simulink model "model"  (R2016b)
settings: Solver=VariableStepAuto  StartTime=0.0  StopTime=4  RelTol=1e-3
undefined symbols (not defined in the file): k1, k2, k_pd, k_pp, k_rp
settings Model: Creator=Kevin K. Kaldvansvik  LastModifiedBy=Kevin K. Kaldvansvik

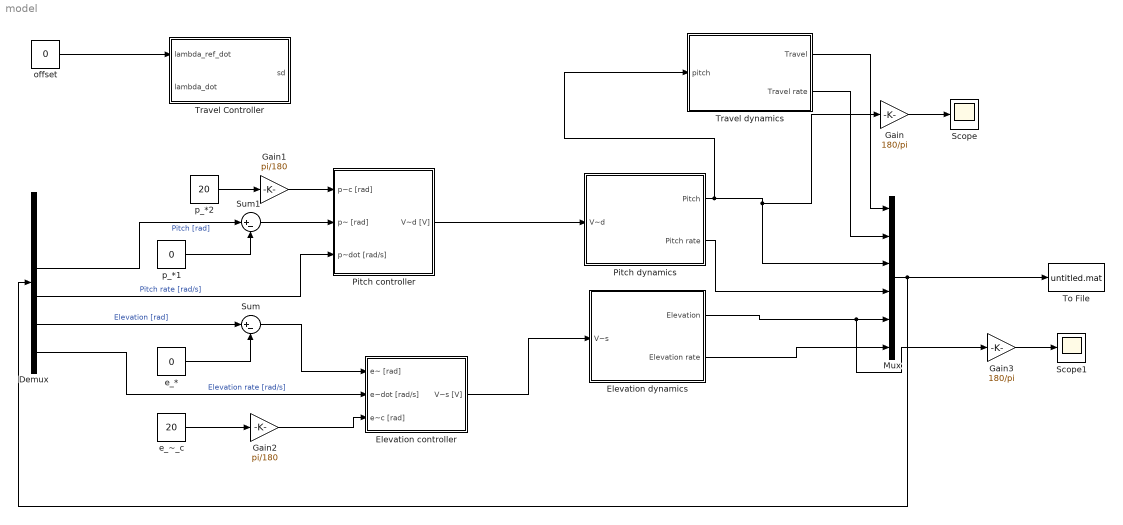
== system model ==
  Demux : Demux  Outputs=6
  Elevation controller : Subsystem
  Elevation dynamics : Subsystem
  Gain : Gain  Gain=180/pi
  Gain1 : Gain  Gain=pi/180
  Gain2 : Gain  Gain=pi/180
  Gain3 : Gain  Gain=180/pi
  Mux : Mux  Inputs=6
  Pitch controller : Subsystem
  Pitch dynamics : Subsystem
  Scope : Scope
  Scope1 : Scope
  Sum : Sum  Inputs=|+-
  Sum1 : Sum  Inputs=|+-
  To File : ToFile  MatrixName=kp_v1
  Travel Controller : Subsystem
  Travel dynamics : Subsystem
  e_* : Constant  Value=0
  e_~_c : Constant  Value=20
  offset : Constant  Value=0
  p_*1 : Constant  Value=0
  p_*2 : Constant  Value=20
  wires:
  e_~_c/1 -> Gain2/1
  e_*/1 -> Sum/2
  Demux/6 -> Elevation controller/2(e~dot [rad/s])  "Elevation rate [rad/s]"
  Sum/1 -> Elevation controller/1(e~ [rad])
  p_*1/1 -> Sum1/2
  Sum1/1 -> Pitch controller/2(p~ [rad])
  Demux/4 -> Pitch controller/3(p~dot [rad/s])  "Pitch rate [rad/s]"
  Mux/1 -> Demux/1, To File/1
  Demux/5 -> Sum/1  "Elevation [rad]"
  Demux/3 -> Sum1/1  "Pitch [rad]"
  offset/1 -> Travel Controller/1("lambda_ref_dot ")
  Pitch controller/1(V~d [V]) -> Pitch dynamics/1(V~d)
  Pitch dynamics/1(Pitch) -> Travel dynamics/1(pitch), Gain/1, Mux/3
  Pitch dynamics/2(Pitch rate) -> Mux/4
  Elevation controller/1(V~s [V]) -> Elevation dynamics/1(V~s)
  Elevation dynamics/1(Elevation) -> Gain3/1, Mux/5
  Elevation dynamics/2(Elevation rate) -> Mux/6
  Travel dynamics/1(Travel) -> Mux/1
  Travel dynamics/2(Travel rate) -> Mux/2
  Gain/1 -> Scope/1
  p_*2/1 -> Gain1/1
  Gain1/1 -> Pitch controller/1(p~c [rad])
  Gain2/1 -> Elevation controller/3(e~c [rad])
  Gain3/1 -> Scope1/1

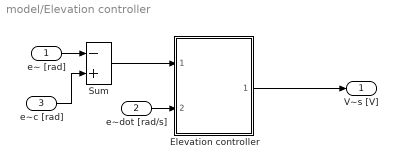
== system model/Elevation controller ==
  e~ [rad] : Inport
  e~dot [rad/s] : Inport  Port=2
  e~c [rad] : Inport  Port=3
  Elevation controller : Subsystem
  Sum : Sum  Inputs=-+  SaturateOnIntegerOverflow=on  InputSameDT=on  OutDataTypeStr=Inherit: Same as first input
  V~s [V] : Outport  InitialOutput=0
  wires:
  Sum/1 -> Elevation controller/1(e~ [rad])
  Elevation controller/1(V~_s [V]) -> V~s [V]/1
  e~ [rad]/1 -> Sum/1
  e~dot [rad/s]/1 -> Elevation controller/2(e~_dot [rad/s])
  e~c [rad]/1 -> Sum/2

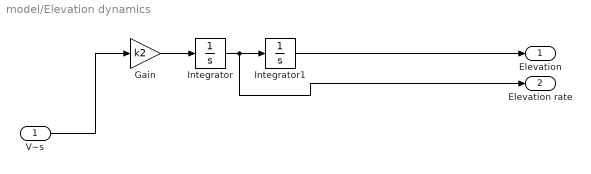
== system model/Elevation dynamics ==
  V~s : Inport
  Gain : Gain  Gain=k2
  Integrator : Integrator
  Integrator1 : Integrator
  Elevation : Outport
  Elevation rate : Outport  Port=2
  wires:
  Gain/1 -> Integrator/1
  Integrator/1 -> Elevation rate/1, Integrator1/1
  V~s/1 -> Gain/1
  Integrator1/1 -> Elevation/1

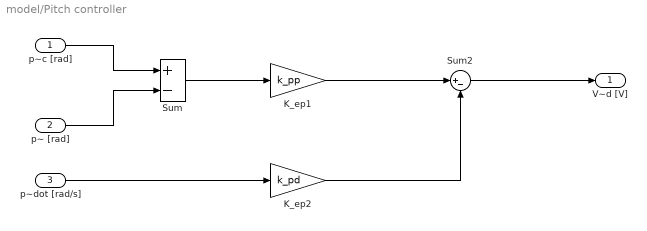
== system model/Pitch controller ==
  p~c [rad] : Inport
  p~ [rad] : Inport  Port=2
  p~dot [rad/s] : Inport  Port=3
  K_ep1 : Gain  Gain=k_pp  SaturateOnIntegerOverflow=on  OutDataTypeStr=Inherit: Same as input  ParamDataTypeStr=Inherit: Same as input
  K_ep2 : Gain  Gain=k_pd  SaturateOnIntegerOverflow=on  OutDataTypeStr=Inherit: Same as input  ParamDataTypeStr=Inherit: Same as input
  Sum : Sum  Inputs=+-  SaturateOnIntegerOverflow=on  InputSameDT=on  OutDataTypeStr=Inherit: Same as first input
  Sum2 : Sum  Inputs=|+-
  V~d [V] : Outport  InitialOutput=0
  wires:
  p~c [rad]/1 -> Sum/1
  p~ [rad]/1 -> Sum/2
  Sum/1 -> K_ep1/1
  p~dot [rad/s]/1 -> K_ep2/1
  K_ep1/1 -> Sum2/1
  K_ep2/1 -> Sum2/2
  Sum2/1 -> V~d [V]/1

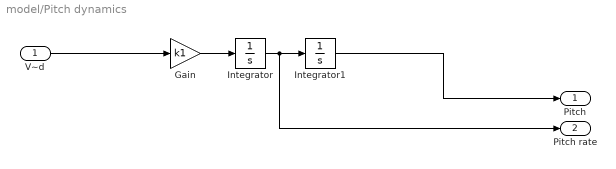
== system model/Pitch dynamics ==
  V~d : Inport
  Gain : Gain  Gain=k1
  Integrator : Integrator
  Integrator1 : Integrator
  Pitch : Outport
  Pitch rate : Outport  Port=2
  wires:
  Integrator/1 -> Pitch rate/1, Integrator1/1
  Integrator1/1 -> Pitch/1
  V~d/1 -> Gain/1
  Gain/1 -> Integrator/1

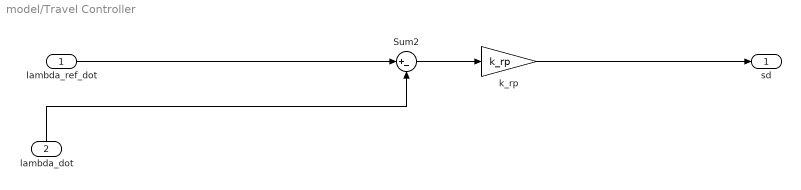
== system model/Travel Controller ==
  "lambda_ref_dot " : Inport
  "lambda_dot " : Inport  Port=2
  Sum2 : Sum  Inputs=|+-
  k_rp : Gain  Gain=k_rp
  "sd " : Outport
  wires:
  k_rp/1 -> "sd "/1
  Sum2/1 -> k_rp/1
  "lambda_ref_dot "/1 -> Sum2/1
  "lambda_dot "/1 -> Sum2/2

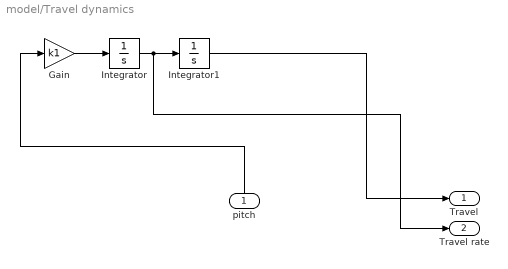
== system model/Travel dynamics ==
  pitch : Inport
  Gain : Gain  Gain=k1
  Integrator : Integrator
  Integrator1 : Integrator
  Travel : Outport
  Travel rate : Outport  Port=2
  wires:
  Gain/1 -> Integrator/1
  Integrator1/1 -> Travel/1
  Integrator/1 -> Travel rate/1, Integrator1/1
  pitch/1 -> Gain/1

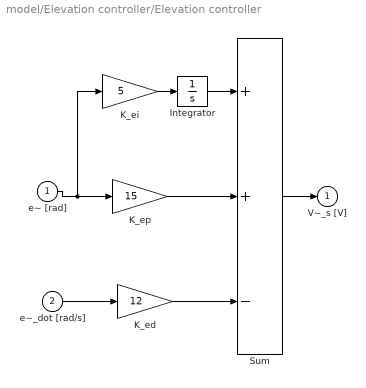
== system model/Elevation controller/Elevation controller ==
  e~ [rad] : Inport
  e~_dot [rad/s] : Inport  Port=2
  Integrator : Integrator  LimitOutput=on
  K_ed : Gain  Gain=12  SaturateOnIntegerOverflow=on  OutDataTypeStr=Inherit: Same as input  ParamDataTypeStr=Inherit: Same as input
  K_ei : Gain  Gain=5  SaturateOnIntegerOverflow=on  OutDataTypeStr=Inherit: Same as input  ParamDataTypeStr=Inherit: Same as input
  K_ep : Gain  Gain=15  SaturateOnIntegerOverflow=on  OutDataTypeStr=Inherit: Same as input  ParamDataTypeStr=Inherit: Same as input
  Sum : Sum  Inputs=++-  SaturateOnIntegerOverflow=on  InputSameDT=on  OutDataTypeStr=Inherit: Same as first input
  V~_s [V] : Outport  InitialOutput=0
  wires:
  K_ei/1 -> Integrator/1
  Integrator/1 -> Sum/1
  Sum/1 -> V~_s [V]/1
  e~_dot [rad/s]/1 -> K_ed/1
  K_ed/1 -> Sum/3
  K_ep/1 -> Sum/2
  e~ [rad]/1 -> K_ep/1, K_ei/1
